simulink model "reactor_final"  (R2025b)
settings: Solver=ode15s  StartTime=0.0  StopTime=10000  RelTol=1e-3
libraries: fl_lib x33, nesl_utility x13, SimscapeFluids_lib x5, ee_lib x1, sdl_lib x1
(part 2 of 2)

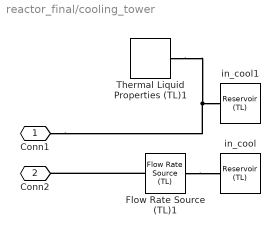
== system reactor_final/cooling_tower ==
  Flow Rate Source (TL)1 : fl_lib/Thermal Liquid/Sources/Flow Rate Source (TL)  source_type=foundation.enum.constant_controlled.constant  flow_type=foundation.enum.mass_volumetric_flow.mass  mass_flow=70000 kg/s  volumetric_flow=0 m^3/s  power_spec=foundation.enum.power_spec.none  area=0.01 m^2
      settings: InternalSimscapePortConfiguration="{\"Bottom\":[],\"Left\":[{\"id\":\"A\",\"label\":\"A\",\"type\":\"foundation.thermal_liquid.thermal_liquid\"}],\"Right\":[{\"id\":\"B\",\"label\":\"B\",\"type\":\"foundation.thermal_liquid.thermal_liquid\"}],\"Top\":[]}"
  Thermal Liquid Properties (TL)1 : SimscapeFluids_lib/Thermal Liquid/Utilities/Thermal Liquid Properties (TL)  fluid_list=fluids.thermal_liquid.utilities.enum.thermal_liquid_fluid_list.water  concentration_param_EG=fluids.thermal_liquid.utilities.enum.thermal_liquid_concentration.volume_fraction  concentration_param_PG=fluids.thermal_liquid.utilities.enum.thermal_liquid_concentration.volume_fraction  c_mass_SW=3.5e-3  c_mass_EG=0.1  c_mass_PG=0.1  c_mass_GL=0.1  c_vol_EG=0.1  c_vol_PG=0.1  beta_const_EG=2.1791 GPa  beta_const_PG=2.1791 GPa  beta_const_GL=2.1791 GPa  p_min_EG=0.01 MPa  p_min_PG=0.01 MPa  p_min_GL=0.01 MPa  p_max_EG=50 MPa  p_max_PG=50 MPa  p_max_GL=50 MPa  p_atm=0.101325 MPa  properties_range_check=simscape.enum.assert.action.error
  in_cool : fl_lib/Thermal Liquid/Elements/Reservoir (TL)  pressure_spec=foundation.enum.pressure_spec.atmospheric  reservoir_pressure=0.1 MPa  reservoir_temperature=290 K  area=0.01 m^2
  in_cool1 : fl_lib/Thermal Liquid/Elements/Reservoir (TL)  pressure_spec=foundation.enum.pressure_spec.atmospheric  reservoir_pressure=0.101325 MPa  reservoir_temperature=290 K  area=2 m^2
  Conn1 : PMIOPort  Side=Left
  Conn2 : PMIOPort  Port=2  Side=Right
  connections:
  Flow Rate Source (TL)1/LConn1 -- in_cool/LConn1
  Thermal Liquid Properties (TL)1/RConn1 -- Conn1/RConn1 -- in_cool1/LConn1
  Flow Rate Source (TL)1/RConn1 -- Conn2/RConn1

== matlab function reactor_final/reactor_core_physics ==
  data: n input; dn_dt output; C input; T_f input; T_c input; rho_ext input; dC_dt output; rho output
function [dn_dt, dC_dt, rho] = reactor_kinetics(n, C, T_f, T_c, rho_ext)
    % U235 Delayed Neutron Data
    lambda = [0.0124; 0.0305; 0.111; 0.301; 1.14; 3.01];
    beta_i = [0.000215; 0.001424; 0.001274; 0.002568; 0.000748; 0.000273];
    beta_total = 0.0065;

    % Reactor Parameters
    Lambda = 1e-4;
    alpha_F = -2.5e-5;
    alpha_C = -1.0e-4;
    
    % Base Reactivity
    T_f_init = 573;
    T_c_init = 600;
    rho_0 = -(alpha_F * T_f_init + alpha_C * T_c_init); 

    rho = rho_0 + rho_ext + (alpha_F * T_f) + (alpha_C * T_c);

    dn_dt = ((rho - beta_total) / Lambda) * n + sum(lambda .* C);

    dC_dt = (beta_i / Lambda) * n - (lambda .* C);
end
